simulink model "torqueBalancingJc_ikin_2012a"  (Simulink 8.0)
settings: Solver=FixedStepDiscrete  StartTime=0.0  StopTime=simulationTime  FixedStep=Ts  RelTol=1e-3
InitFcn:
  | initTorqueBalancingJc;
values from neighbouring files (symbols this model uses):
  LEFT_RIGHT_FOOT_IN_CONTACT = [1 1]    [initTorqueBalancingJc.m]
  localName = 'matlabTorqueBalancing'    [initTorqueBalancingJc.m]
  Ts = 0.01    [initTorqueBalancingJc.m]
undefined symbols (not defined in the file or in its folder): bVectorConstraints, ConstraintsMatrix, DiscIntNeverNeededParam, gain, reg, ROBOT_DOF, ROBOT_DOF_FOR_SIMULINK, sat
undefined symbols (not defined in the file): robotName
libraries: WBCLibrary x57, simulink x2
settings Model: Creator=daniele  LastModifiedBy=jorhabib
settings DebuggingCC: FcnCallInpInsideContextMsg=EnableAllAsWarning  FrameProcessingCompatibilityMsg=error
settings SFSimCC: SimParseCustomCode=off
settings CodeAppCC: CustomSymbolStrType=$N$R$M_T
settings GRTTargetCC: CodeReplacementLibrary=C89/C90 (ANSI)  CombineOutputUpdateFcns=off  GRTInterface=on

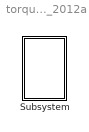
== system torqueBalancingJc_ikin_2012a ==
  Subsystem : Subsystem  mask{robotName=robotName, Ts=Ts, localName=localName}
      mask prompts: robotName "robot name"; localName "module name"

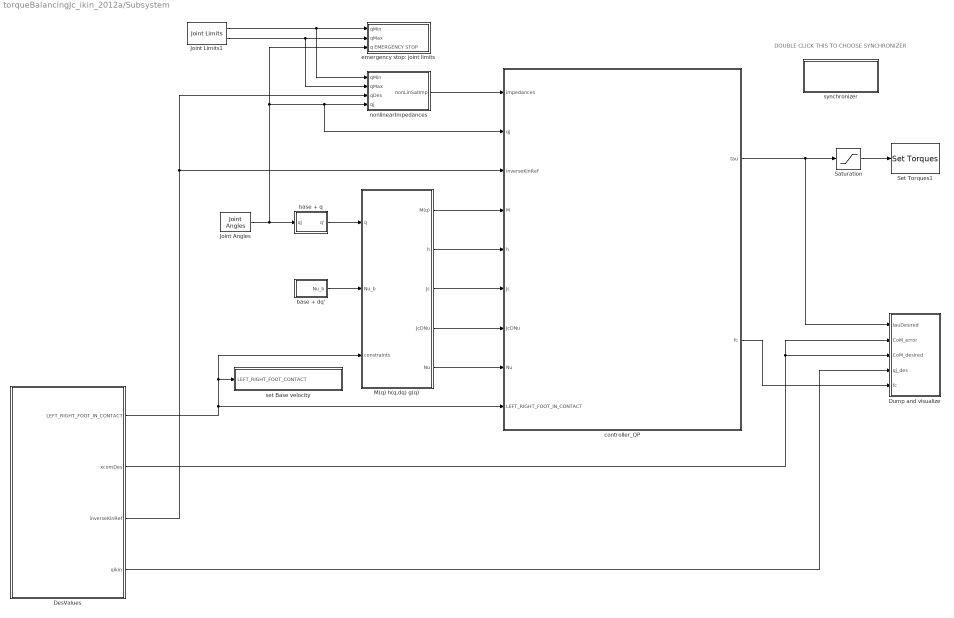
== system torqueBalancingJc_ikin_2012a/Subsystem ==
  note: DOUBLE CLICK THIS TO
      |  CHOOSE SYNCHRONIZER
  DesValues : Subsystem
  Dump and visualize : Subsystem
  Joint Angles : WBCLibrary/wholeBodyStates/Joint Angles  robotName=robotName  localName=localName
  Joint Limits1 : WBCLibrary/wholeBodyModel/Joint Limits  robotName=robotName  localName=localName
  M(q) h(q,dq) g(q) : Subsystem
  Saturation : Saturate  UpperLimit=sat.torque  LowerLimit=-sat.torque
  Set Torques1 : WBCLibrary/wholeBodyActuators/Set Torques  val=6  robotName=robotName  localName=localName
  base + dq' : Subsystem
  base + q : Subsystem
  controller_QP : Subsystem
  emergency stop: joint limits : Subsystem
  nonlinearImpedances : Subsystem
  set Base velocity : Subsystem  Description=Set base velocity
  synchronizer : Subsystem
  wires:
  base + q/1(q') -> M(q) h(q,dq) g(q)/1(q)
  M(q) h(q,dq) g(q)/1(M(q)) -> controller_QP/4(M)
  Joint Limits1/1 -> emergency stop: joint limits/1(qMin), nonlinearImpedances/1(qMin)
  Joint Limits1/2 -> emergency stop: joint limits/2(qMax), nonlinearImpedances/2(qMax)
  Joint Angles/1 -> emergency stop: joint limits/3(q EMERGENCY STOP), controller_QP/2(qj), nonlinearImpedances/4(qj), base + q/1(qj)
  M(q) h(q,dq) g(q)/2(h) -> controller_QP/5(h)
  controller_QP/1("tau ") -> Dump and visualize/1(tauDesired), Saturation/1
  Saturation/1 -> Set Torques1/1
  DesValues/1(LEFT_RIGHT_FOOT_IN_CONTACT) -> M(q) h(q,dq) g(q)/3(constraints), set Base velocity/1(LEFT_RIGHT_FOOT_CONTACT), controller_QP/9(LEFT_RIGHT_FOOT_IN_CONTACT)
  nonlinearImpedances/1(nonLinSatImp) -> controller_QP/1(impedances)
  M(q) h(q,dq) g(q)/5(Nu) -> controller_QP/8(Nu)
  M(q) h(q,dq) g(q)/3(Jc) -> controller_QP/6(Jc)
  M(q) h(q,dq) g(q)/4(JcDNu) -> controller_QP/7(JcDNu)
  DesValues/3(inverseKinRef) -> controller_QP/3(inverseKinRef), nonlinearImpedances/3(qDes)
  base + dq'/1(Nu_b) -> M(q) h(q,dq) g(q)/2(Nu_b)
  DesValues/4(qikin) -> Dump and visualize/4(qj_des)
  DesValues/2(xcomDes) -> Dump and visualize/2(CoM_error), Dump and visualize/3(CoM_desired)
  controller_QP/2(fc) -> Dump and visualize/5(fc)

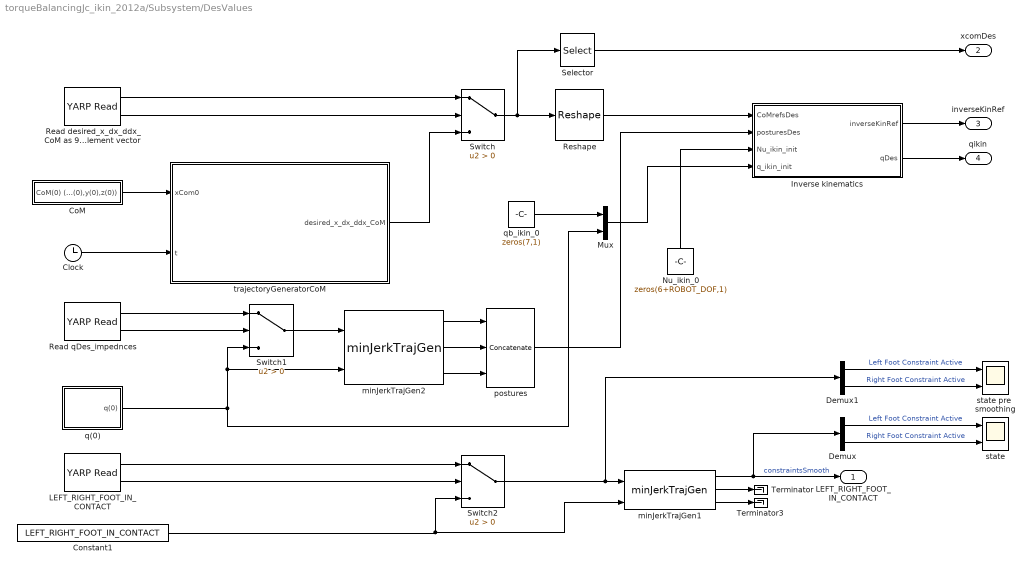
== system torqueBalancingJc_ikin_2012a/Subsystem/DesValues ==
  " LEFT_RIGHT_FOOT_IN_CONTACT" : WBCLibrary/Utilities/YARP Read  portName=['/' localName '/constraints:i']  signalSize=2  blocking=off  timestamp=off  autoconnect=off  errorOnConnection=on
  Clock : Clock
  "CoM " : Subsystem
  Constant1 : Constant  Value=LEFT_RIGHT_FOOT_IN_CONTACT
  Demux : Demux  Outputs=2
  Demux1 : Demux  Outputs=2
  Inverse kinematics : Subsystem
  Mux : Mux  Inputs=2
  Nu_ikin_0 : Constant  Value=zeros(6+ROBOT_DOF,1)
  "Read desired_x_dx_ddx_CoM as 9 element vector " : WBCLibrary/Utilities/YARP Read  portName=['/' localName '/comDes:i']  signalSize=9  blocking=off  timestamp=off  autoconnect=off  errorOnConnection=on
  Read qDes_impednces : WBCLibrary/Utilities/YARP Read  portName=['/' localName '/qDes:i']  signalSize=ROBOT_DOF  blocking=off  timestamp=off  autoconnect=off  errorOnConnection=on
  Reshape : Reshape  OutputDimensionality=Customize  OutputDimensions=[3,3]
  Selector : Selector  InputPortWidth=9  IndexOptions=Index vector (dialog)  Indices=[1:3]  OutputSizes=1
  Switch : Switch  Criteria=u2 > Threshold
  Switch1 : Switch  Criteria=u2 > Threshold
  Switch2 : Switch  Criteria=u2 > Threshold
  Terminator : Terminator
  Terminator3 : Terminator
  minJerkTrajGen1 : WBCLibrary/Utilities/minJerkTrajGen  dim=2  Ts=Ts  Tt=smoothingTimeJacobians
  minJerkTrajGen2 : WBCLibrary/Utilities/minJerkTrajGen  dim=ROBOT_DOF  Ts=Ts  Tt=smoothingTimePostures
  postures : Concatenate  NumInputs=3  Mode=Multidimensional array  ConcatenateDimension=2
  q(0) : Subsystem
  qb_ikin_0 : Constant  Value=zeros(7,1)
  state : Scope  NumInputPorts=2
      settings: ShowLegends=on  TimeRange=60  YMin=0~0  YMax=2~2
  state pre  smoothing : Scope  NumInputPorts=2
      settings: ShowLegends=on  TimeRange=60  YMin=0~0  YMax=2~2  SaveName=ScopeData7
  trajectoryGeneratorCoM : MATLAB Function  TreatAsAtomicUnit=on
  LEFT_RIGHT_FOOT_IN_CONTACT : Outport
  xcomDes : Outport  Port=2
  inverseKinRef : Outport  Port=3
  qikin : Outport  Port=4
  wires:
  Constant1/1 -> Switch2/3, minJerkTrajGen1/2
  minJerkTrajGen1/1 -> Demux/1, LEFT_RIGHT_FOOT_IN_CONTACT/1  "constraintsSmooth"
  minJerkTrajGen1/2 -> Terminator/1
  minJerkTrajGen1/3 -> Terminator3/1
  "Read desired_x_dx_ddx_CoM as 9 element vector "/2 -> Switch/2
  "Read desired_x_dx_ddx_CoM as 9 element vector "/1 -> Switch/1
  Reshape/1 -> Inverse kinematics/1(CoMrefsDes)
  Switch/1 -> Selector/1, Reshape/1
  Read qDes_impednces/2 -> Switch1/2
  Read qDes_impednces/1 -> Switch1/1
  Selector/1 -> xcomDes/1
  " LEFT_RIGHT_FOOT_IN_CONTACT"/2 -> Switch2/2
  " LEFT_RIGHT_FOOT_IN_CONTACT"/1 -> Switch2/1
  Switch2/1 -> Demux1/1, minJerkTrajGen1/1
  Demux/1 -> state/1  "Left Foot Constraint Active"
  Demux/2 -> state/2  "Right Foot Constraint Active"
  Demux1/1 -> state pre  smoothing/1  "Left Foot Constraint Active"
  Demux1/2 -> state pre  smoothing/2  "Right Foot Constraint Active"
  "CoM "/1(CoM(0) (x(0),y(0),z(0))) -> trajectoryGeneratorCoM/1(xCom0)
  Clock/1 -> trajectoryGeneratorCoM/2(t)
  trajectoryGeneratorCoM/1(desired_x_dx_ddx_CoM) -> Switch/3
  Switch1/1 -> minJerkTrajGen2/1
  minJerkTrajGen2/1 -> postures/1
  minJerkTrajGen2/2 -> postures/2
  minJerkTrajGen2/3 -> postures/3
  Nu_ikin_0/1 -> Inverse kinematics/3(Nu_ikin_init)
  qb_ikin_0/1 -> Mux/1
  Mux/1 -> Inverse kinematics/4(q_ikin_init)
  q(0)/1(q(0)) -> Mux/2, Switch1/3, minJerkTrajGen2/2
  Inverse kinematics/1(inverseKinRef) -> inverseKinRef/1
  postures/1 -> Inverse kinematics/2(posturesDes)
  Inverse kinematics/2(qDes) -> qikin/1

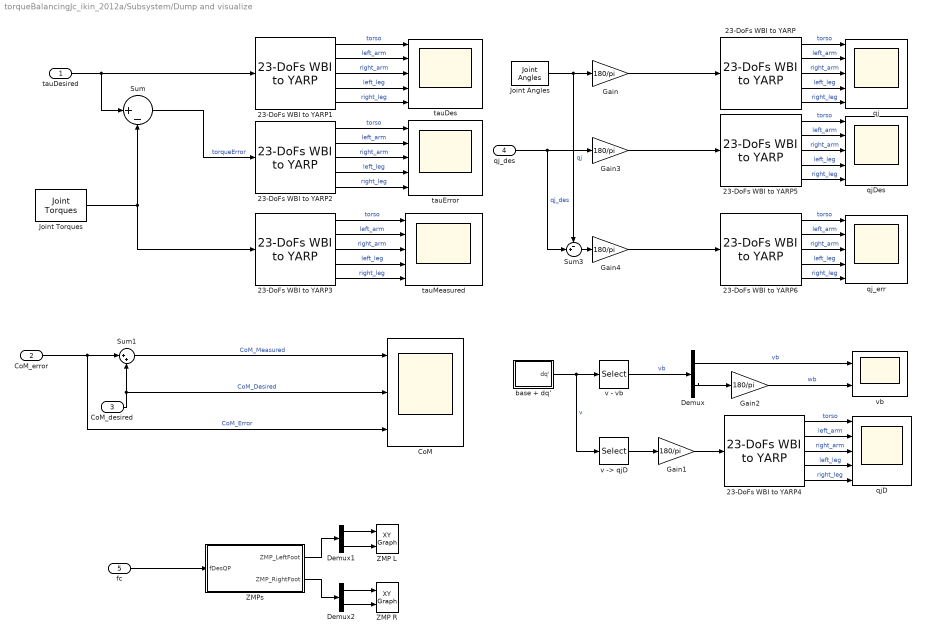
== system torqueBalancingJc_ikin_2012a/Subsystem/Dump and visualize ==
  tauDesired : Inport
  CoM_error : Inport  Port=2
  CoM_desired : Inport  Port=3
  qj_des : Inport  Port=4
  fc : Inport  Port=5
  23-DoFs WBI to YARP{,1..6} (7 alike) : WBCLibrary/Utilities/23-DoFs WBI to YARP
  CoM : Scope  NumInputPorts=3
      settings: ShowLegends=on  TimeRange=400  YMin=-0.2~-0.2~-0.006  YMax=0.5~0.5~0.004  SaveName=CoM_data
  Demux : Demux  Outputs=2
  Demux1 : Demux  Outputs=2
  Demux2 : Demux  Outputs=2
  Gain{,1..4} (5 alike) : Gain  Gain=180/pi
  Joint Angles : WBCLibrary/wholeBodyStates/Joint Angles  robotName=robotName  localName=localName
  Joint Torques : WBCLibrary/wholeBodyStates/Joint Torques  robotName=robotName  localName=localName
  Sum : Sum  Inputs=|+-
  Sum1 : Sum  Inputs=|++
  Sum3 : Sum  Inputs=-+|
  ZMP L : simulink/Sinks/XY Graph  xmin=gain.footSize(1,1)  xmax=gain.footSize(1,2)  ymin=gain.footSize(2,1)  ymax=gain.footSize(2,2)  st=-1
  ZMP R : simulink/Sinks/XY Graph  xmin=gain.footSize(1,1)  xmax=gain.footSize(1,2)  ymin=gain.footSize(2,1)  ymax=gain.footSize(2,2)  st=-1
  ZMPs : Subsystem
  base + dq' : Subsystem
  qj : Scope  NumInputPorts=5
      settings: ShowLegends=on  TimeRange=40  YMin=-6~-40~-40~-15~-10  YMax=2~60~60~15~12.5  SaveName=qj_and_v
  qjD : Scope  NumInputPorts=5
      settings: ShowLegends=on  TimeRange=40  YMin=-15~-10~-20~-20~-20  YMax=20~10~30~20~20  SaveName=qj_and_v1
  qjDes : Scope  NumInputPorts=5
      settings: ShowLegends=on  TimeRange=40  YMin=-6~-40~-40~-15~-10  YMax=2~60~60~15~12.5  SaveName=qj_and_v3
  qj_err : Scope  NumInputPorts=5
      settings: ShowLegends=on  TimeRange=40  YMin=-0.05~-0.01~-0.015~-0.25~-0.5  YMax=0.125~0.02~0.02~1.25~2.5  SaveName=qj_and_v4
  tauDes : Scope  NumInputPorts=5
      settings: ShowLegends=on  TimeRange=14  YMin=-5~-2.5~-2.5~-4~-3.5  YMax=1~1.5~1.5~3~2  SaveName=tauDes
  tauError : Scope  NumInputPorts=5
      settings: ShowLegends=on  TimeRange=90  YMin=-3.94704~-2.86095~-2.77437~-5.99629~-4.78678  YMax=3.1474~3.19748~2.86308~6.73695~4.3906  SaveName=tauError
  tauMeasured : Scope  NumInputPorts=5
      settings: ShowLegends=on  TimeRange=14  YMin=-800000~-300000~-300000~-500000~-1e+06  YMax=100000~200000~200000~600000~1e+06  SaveName=tauMeasured
  v - vb : Selector  InputPortWidth=ROBOT_DOF+6  IndexOptions=Index vector (dialog)  Indices=[1:6]  OutputSizes=1
  "v -> qjD" : Selector  InputPortWidth=ROBOT_DOF+6  IndexOptions=Index vector (dialog)  Indices=[7:ROBOT_DOF+6]  OutputSizes=1
  vb : Scope  NumInputPorts=2
      settings: ShowLegends=on  TimeRange=40  YMin=-0.08~-10  YMax=0.08~10  SaveName=qj_and_v2
  wires:
  CoM_error/1 -> CoM/3, Sum1/1  "CoM_Error"
  CoM_desired/1 -> Sum1/2, CoM/2  "CoM_Desired"
  Sum1/1 -> CoM/1  "CoM_Measured"
  base + dq'/1(dq') -> "v -> qjD"/1, v - vb/1  "v"
  Joint Angles/1 -> Sum3/1, Gain/1  "qj"
  Gain/1 -> 23-DoFs WBI to YARP/1
  23-DoFs WBI to YARP/5 -> qj/5  "right_leg"
  23-DoFs WBI to YARP/1 -> qj/1  "torso"
  23-DoFs WBI to YARP/2 -> qj/2  "left_arm"
  23-DoFs WBI to YARP/4 -> qj/4  "left_leg"
  23-DoFs WBI to YARP/3 -> qj/3  "right_arm"
  23-DoFs WBI to YARP4/5 -> qjD/5  "right_leg"
  23-DoFs WBI to YARP4/1 -> qjD/1  "torso"
  23-DoFs WBI to YARP4/2 -> qjD/2  "left_arm"
  23-DoFs WBI to YARP4/4 -> qjD/4  "left_leg"
  23-DoFs WBI to YARP4/3 -> qjD/3  "right_arm"
  "v -> qjD"/1 -> Gain1/1
  v - vb/1 -> Demux/1  "vb"
  Demux/1 -> vb/1  "vb"
  Demux/2 -> Gain2/1
  Gain1/1 -> 23-DoFs WBI to YARP4/1
  Gain2/1 -> vb/2  "wb"
  fc/1 -> ZMPs/1(fDesQP)
  ZMPs/1(ZMP_LeftFoot) -> Demux1/1
  ZMPs/2(ZMP_RightFoot) -> Demux2/1
  Demux1/1 -> ZMP L/1
  Demux1/2 -> ZMP L/2
  Demux2/1 -> ZMP R/1
  Demux2/2 -> ZMP R/2
  tauDesired/1 -> Sum/1, 23-DoFs WBI to YARP1/1
  Joint Torques/1 -> 23-DoFs WBI to YARP3/1, Sum/2
  23-DoFs WBI to YARP1/5 -> tauDes/5  "right_leg"
  23-DoFs WBI to YARP1/1 -> tauDes/1  "torso"
  23-DoFs WBI to YARP1/2 -> tauDes/2  "left_arm"
  23-DoFs WBI to YARP1/4 -> tauDes/4  "left_leg"
  23-DoFs WBI to YARP1/3 -> tauDes/3  "right_arm"
  23-DoFs WBI to YARP2/5 -> tauError/5  "right_leg"
  23-DoFs WBI to YARP2/1 -> tauError/1  "torso"
  23-DoFs WBI to YARP2/2 -> tauError/2  "left_arm"
  23-DoFs WBI to YARP2/4 -> tauError/4  "left_leg"
  23-DoFs WBI to YARP2/3 -> tauError/3  "right_arm"
  Sum/1 -> 23-DoFs WBI to YARP2/1  "torqueError"
  23-DoFs WBI to YARP3/5 -> tauMeasured/5  "right_leg"
  23-DoFs WBI to YARP3/1 -> tauMeasured/1  "torso"
  23-DoFs WBI to YARP3/2 -> tauMeasured/2  "left_arm"
  23-DoFs WBI to YARP3/4 -> tauMeasured/4  "left_leg"
  23-DoFs WBI to YARP3/3 -> tauMeasured/3  "right_arm"
  Gain3/1 -> 23-DoFs WBI to YARP5/1
  23-DoFs WBI to YARP5/5 -> qjDes/5  "right_leg"
  23-DoFs WBI to YARP5/1 -> qjDes/1  "torso"
  23-DoFs WBI to YARP5/2 -> qjDes/2  "left_arm"
  23-DoFs WBI to YARP5/4 -> qjDes/4  "left_leg"
  23-DoFs WBI to YARP5/3 -> qjDes/3  "right_arm"
  Gain4/1 -> 23-DoFs WBI to YARP6/1
  23-DoFs WBI to YARP6/5 -> qj_err/5  "right_leg"
  23-DoFs WBI to YARP6/1 -> qj_err/1  "torso"
  23-DoFs WBI to YARP6/2 -> qj_err/2  "left_arm"
  23-DoFs WBI to YARP6/4 -> qj_err/4  "left_leg"
  23-DoFs WBI to YARP6/3 -> qj_err/3  "right_arm"
  Sum3/1 -> Gain4/1
  qj_des/1 -> Gain3/1, Sum3/2  "qj_des"

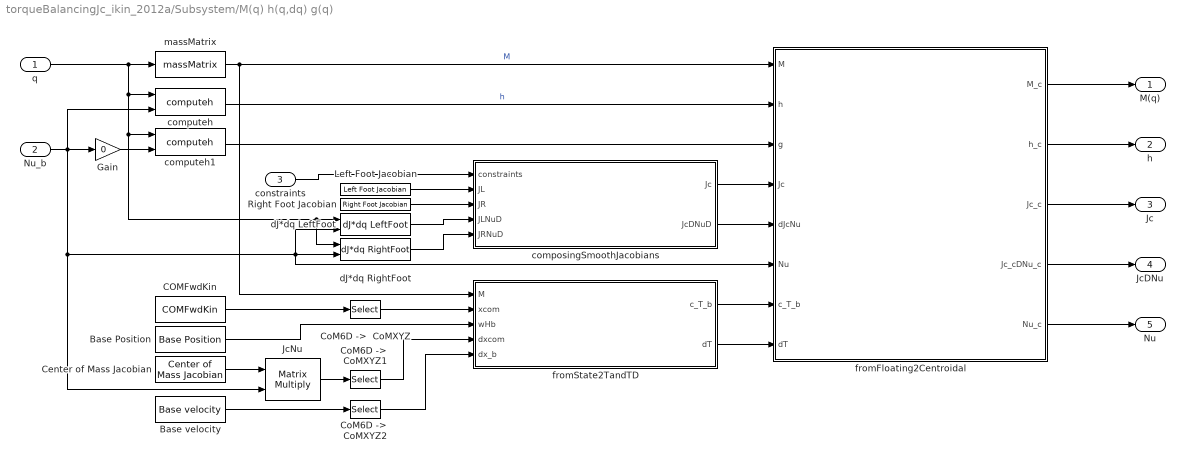
== system torqueBalancingJc_ikin_2012a/Subsystem/M(q) h(q,dq) g(q) ==
  q : Inport
  Nu_b : Inport  Port=2
  constraints : Inport  Port=3
  Base Position : WBCLibrary/wholeBodyStates/Base Position  robotName=robotName  localName=localName
  Base velocity : WBCLibrary/wholeBodyStates/Base velocity  robotName=robotName  localName=localName
  "COMFwdKin " : WBCLibrary/wholeBodyModel/Forward Kinematics/COMFwdKin   robotName=robotName  localName=localName
  Center of Mass Jacobian : WBCLibrary/wholeBodyModel/Jacobians/Center of Mass Jacobian  robotName=robotName  localName=localName
  "CoM6D ->  CoMXYZ" : Selector  InputPortWidth=7  IndexOptions=Index vector (dialog)  Indices=[1 2 3]  OutputSizes=1
  "CoM6D ->  CoMXYZ1" : Selector  InputPortWidth=6  IndexOptions=Index vector (dialog)  Indices=[1 2 3]  OutputSizes=1
  "CoM6D ->  CoMXYZ2" : Selector  InputPortWidth=6  IndexOptions=Index vector (dialog)  Indices=[1 2 3]  OutputSizes=1
  Gain : Gain  Gain=0
  JcNu : Product  Multiplication=Matrix(*)
  Left Foot Jacobian : WBCLibrary/wholeBodyModel/Jacobians/Left Foot Jacobian  robotName=robotName  localName=localName
  Right Foot Jacobian : WBCLibrary/wholeBodyModel/Jacobians/Right Foot Jacobian  robotName=robotName  localName=localName
  composingSmoothJacobians : MATLAB Function  TreatAsAtomicUnit=on
  computeh : WBCLibrary/wholeBodyModel/Dynamics/computeh  val=7  robotname=robotName  localname=localName
  computeh1 : WBCLibrary/wholeBodyModel/Dynamics/computeh  val=7  robotname=robotName  localname=localName
  dJ*dq LeftFoot : WBCLibrary/wholeBodyModel/Dynamics/dJ*dq LeftFoot  val=9  robotName=robotName  localName=localName
  dJ*dq RightFoot : WBCLibrary/wholeBodyModel/Dynamics/dJ*dq RightFoot  val=9  robotName=robotName  localName=localName
  fromFloating2Centroidal : MATLAB Function  TreatAsAtomicUnit=on
  fromState2TandTD : MATLAB Function  TreatAsAtomicUnit=on
  massMatrix : WBCLibrary/wholeBodyModel/Dynamics/massMatrix  val=8  robotname=robotName  localname=localName
  M(q) : Outport
  h : Outport  Port=2
  Jc : Outport  Port=3
  JcDNu : Outport  Port=4
  Nu : Outport  Port=5
  wires:
  q/1 -> computeh1/1, dJ*dq RightFoot/1, dJ*dq LeftFoot/1, computeh/1, massMatrix/1
  Nu_b/1 -> Gain/1, computeh/2, fromFloating2Centroidal/6(Nu), dJ*dq LeftFoot/2, dJ*dq RightFoot/2, JcNu/2
  Gain/1 -> computeh1/2
  massMatrix/1 -> fromFloating2Centroidal/1(M), fromState2TandTD/1(M)  "M"
  fromState2TandTD/1(c_T_b) -> fromFloating2Centroidal/7(c_T_b)
  fromState2TandTD/2(dT) -> fromFloating2Centroidal/8(dT)
  computeh/1 -> fromFloating2Centroidal/2(h)  "h"
  computeh1/1 -> fromFloating2Centroidal/3(g)
  "COMFwdKin "/1 -> "CoM6D ->  CoMXYZ"/1
  "CoM6D ->  CoMXYZ"/1 -> fromState2TandTD/2(xcom)
  Base velocity/1 -> "CoM6D ->  CoMXYZ2"/1
  "CoM6D ->  CoMXYZ2"/1 -> fromState2TandTD/5(dx_b)
  Base Position/1 -> fromState2TandTD/3(wHb)
  Center of Mass Jacobian/1 -> JcNu/1
  JcNu/1 -> "CoM6D ->  CoMXYZ1"/1
  "CoM6D ->  CoMXYZ1"/1 -> fromState2TandTD/4(dxcom)
  composingSmoothJacobians/1(Jc) -> fromFloating2Centroidal/4(Jc)
  composingSmoothJacobians/2(JcDNuD) -> fromFloating2Centroidal/5(dJcNu)
  constraints/1 -> composingSmoothJacobians/1(constraints)
  Left Foot Jacobian/1 -> composingSmoothJacobians/2(JL)
  Right Foot Jacobian/1 -> composingSmoothJacobians/3(JR)
  dJ*dq LeftFoot/1 -> composingSmoothJacobians/4(JLNuD)
  dJ*dq RightFoot/1 -> composingSmoothJacobians/5(JRNuD)
  fromFloating2Centroidal/1(M_c) -> M(q)/1
  fromFloating2Centroidal/2(h_c) -> h/1
  fromFloating2Centroidal/3(Jc_c) -> Jc/1
  fromFloating2Centroidal/4(Jc_cDNu_c) -> JcDNu/1
  fromFloating2Centroidal/5(Nu_c) -> Nu/1

== system torqueBalancingJc_ikin_2012a/Subsystem/base + dq' ==
  Base velocity : WBCLibrary/wholeBodyStates/Base velocity  robotName=robotName  localName=localName
  Joint Velocities : WBCLibrary/wholeBodyStates/Joint Velocities  robotName=robotName  localName=localName
  Mux : Mux  Inputs=2
  Nu_b : Outport
  wires:
  Base velocity/1 -> Mux/1
  Joint Velocities/1 -> Mux/2
  Mux/1 -> Nu_b/1

== system torqueBalancingJc_ikin_2012a/Subsystem/base + q ==
  qj : Inport
  Constant1 : Constant  Value=zeros(16,1)
  Mux : Mux  Inputs=2
  q' : Outport
  wires:
  Mux/1 -> q'/1
  qj/1 -> Mux/2
  Constant1/1 -> Mux/1

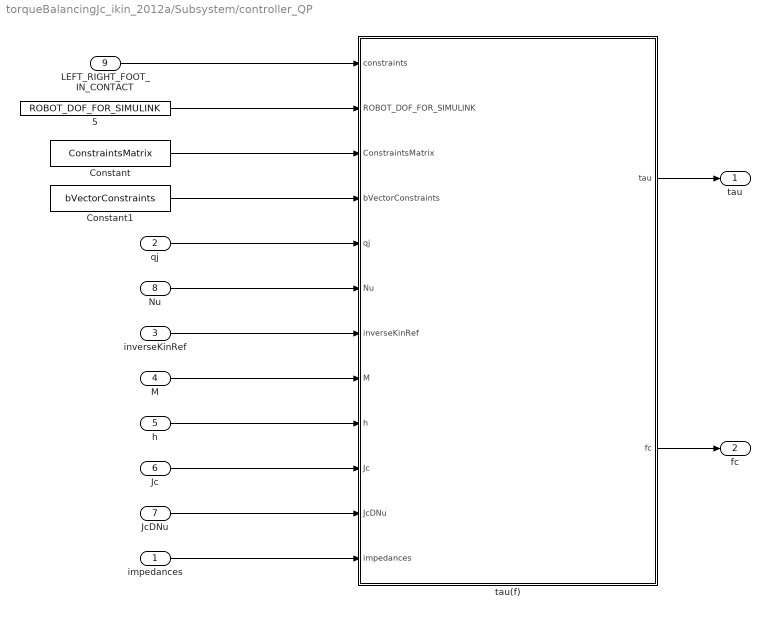
== system torqueBalancingJc_ikin_2012a/Subsystem/controller_QP ==
  impedances : Inport
  qj : Inport  Port=2
  inverseKinRef : Inport  Port=3
  M : Inport  Port=4
  h : Inport  Port=5
  Jc : Inport  Port=6
  JcDNu : Inport  Port=7
  Nu : Inport  Port=8
  LEFT_RIGHT_FOOT_IN_CONTACT : Inport  Port=9
  "    5" : Constant  Value=ROBOT_DOF_FOR_SIMULINK
  Constant : Constant  Value=ConstraintsMatrix
  Constant1 : Constant  Value=bVectorConstraints
  "tau(f) " : MATLAB Function  TreatAsAtomicUnit=on
  "tau " : Outport
  fc : Outport  Port=2
  wires:
  LEFT_RIGHT_FOOT_IN_CONTACT/1 -> "tau(f) "/1(constraints)
  M/1 -> "tau(f) "/8(M)
  h/1 -> "tau(f) "/9(h)
  "    5"/1 -> "tau(f) "/2(ROBOT_DOF_FOR_SIMULINK)
  Constant/1 -> "tau(f) "/3(ConstraintsMatrix)
  Constant1/1 -> "tau(f) "/4(bVectorConstraints)
  Jc/1 -> "tau(f) "/10(Jc)
  JcDNu/1 -> "tau(f) "/11(JcDNu)
  Nu/1 -> "tau(f) "/6(Nu)
  impedances/1 -> "tau(f) "/12(impedances)
  "tau(f) "/1(tau) -> "tau "/1
  qj/1 -> "tau(f) "/5(qj)
  inverseKinRef/1 -> "tau(f) "/7(inverseKinRef)
  "tau(f) "/2(fc) -> fc/1

== system torqueBalancingJc_ikin_2012a/Subsystem/emergency stop: joint limits ==
  qMin : Inport
  qMax : Inport  Port=2
  q EMERGENCY STOP : Inport  Port=3
  Assertion : Assertion  Enabled=on
  MATLAB Function : MATLAB Function  TreatAsAtomicUnit=on
  index1 : Constant  Value=0.01  VectorParams1D=off
  wires:
  qMin/1 -> MATLAB Function/1(umin)
  qMax/1 -> MATLAB Function/2(umax)
  index1/1 -> MATLAB Function/4(tol)
  q EMERGENCY STOP/1 -> MATLAB Function/3(u)
  MATLAB Function/1(inRange) -> Assertion/1

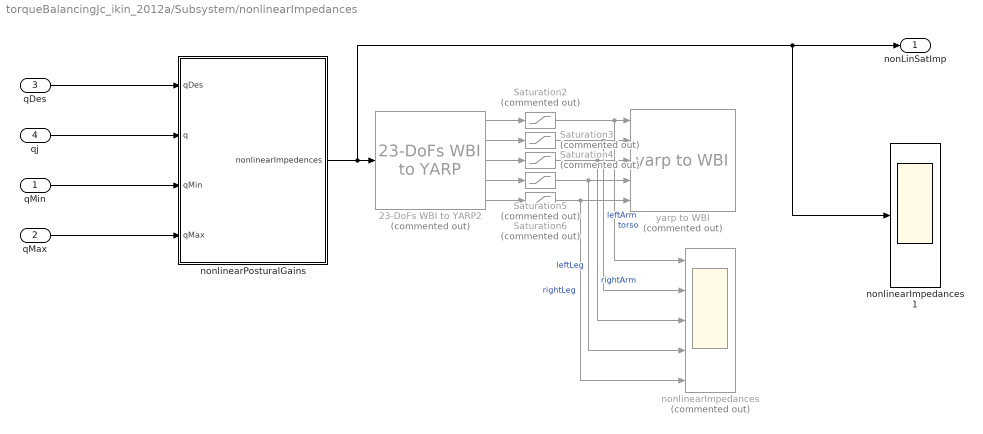
== system torqueBalancingJc_ikin_2012a/Subsystem/nonlinearImpedances ==
  qMin : Inport
  qMax : Inport  Port=2
  qDes : Inport  Port=3
  qj : Inport  Port=4
  23-DoFs WBI to YARP2 : WBCLibrary/Utilities/23-DoFs WBI to YARP  Commented=on
  Saturation2 : Saturate  Commented=on  UpperLimit=sat.impedences(1)  LowerLimit=0  SampleTime=Ts
  Saturation3 : Saturate  Commented=on  UpperLimit=sat.impedences(2)  LowerLimit=0  SampleTime=Ts
  Saturation4 : Saturate  Commented=on  UpperLimit=sat.impedences(2)  LowerLimit=0  SampleTime=Ts
  Saturation5 : Saturate  Commented=on  UpperLimit=sat.impedences(3)  LowerLimit=0  SampleTime=Ts
  Saturation6 : Saturate  Commented=on  UpperLimit=sat.impedences(3)  LowerLimit=0  SampleTime=Ts
  nonlinearImpedances : Scope  Commented=on  NumInputPorts=5
      settings: ShowLegends=on  TimeRange=25  YMin=-50~-50~-50~0~0  YMax=50~50~50~1000~1000
  nonlinearImpedances1 : Scope
      settings: ShowLegends=on  TimeRange=25  YMin=-50  YMax=50
  "nonlinearPosturalGains " : MATLAB Function  TreatAsAtomicUnit=on
  yarp to WBI : WBCLibrary/Utilities/yarp to WBI  Commented=on
  nonLinSatImp : Outport
  wires:
  23-DoFs WBI to YARP2/1 -> Saturation2/1
  23-DoFs WBI to YARP2/2 -> Saturation3/1
  23-DoFs WBI to YARP2/3 -> Saturation4/1
  23-DoFs WBI to YARP2/5 -> Saturation6/1
  "nonlinearPosturalGains "/1(nonlinearImpedences) -> nonlinearImpedances1/1, nonLinSatImp/1, 23-DoFs WBI to YARP2/1
  qMin/1 -> "nonlinearPosturalGains "/3(qMin)
  qMax/1 -> "nonlinearPosturalGains "/4(qMax)
  qj/1 -> "nonlinearPosturalGains "/2(q)
  Saturation6/1 -> nonlinearImpedances/5, yarp to WBI/5  "rightLeg"
  Saturation4/1 -> nonlinearImpedances/3, yarp to WBI/3  "rightArm"
  Saturation5/1 -> nonlinearImpedances/4, yarp to WBI/4  "leftLeg"
  Saturation3/1 -> nonlinearImpedances/2, yarp to WBI/2  "leftArm"
  Saturation2/1 -> nonlinearImpedances/1, yarp to WBI/1  "torso"
  23-DoFs WBI to YARP2/4 -> Saturation5/1
  qDes/1 -> "nonlinearPosturalGains "/1(qDes)

== system torqueBalancingJc_ikin_2012a/Subsystem/set Base velocity ==
  LEFT_RIGHT_FOOT_CONTACT : Inport
  Joint Velocities : WBCLibrary/wholeBodyStates/Joint Velocities  robotName=robotName  localName=localName
  Left Foot Jacobian : WBCLibrary/wholeBodyModel/Jacobians/Left Foot Jacobian  robotName=robotName  localName=localName
  Right Foot Jacobian : WBCLibrary/wholeBodyModel/Jacobians/Right Foot Jacobian  robotName=robotName  localName=localName
  Set base velocity (w.r.t. world) : WBCLibrary/wholeBodyStates/Set base velocity (w.r.t. world)  Priority=-1  robotName=robotName  localName=localName
  baseVelocity : Subsystem  AncestorBlock=WBCLibrary/Utilities/baseVelocity  mask(baseVelocity){}
      mask help: This block computes the velocity of the floating base of a bipedal robot
  wires:
  Left Foot Jacobian/1 -> baseVelocity/2(JacobLF)
  Right Foot Jacobian/1 -> baseVelocity/1(JacobRF)
  baseVelocity/1(baseVel) -> Set base velocity (w.r.t. world)/1
  Joint Velocities/1 -> baseVelocity/3(dq)
  LEFT_RIGHT_FOOT_CONTACT/1 -> baseVelocity/4(LEFT_RIGHT_FOOT_CONTACT)

== system torqueBalancingJc_ikin_2012a/Subsystem/synchronizer ==
  Real Time Synchronizer : WBCLibrary/Utilities/Real Time Synchronizer  Commented=on  threadPeriod=Ts
  synchronize : WBCLibrary/Utilities/synchronize  rate=0.010  scaleFactor=1

== system torqueBalancingJc_ikin_2012a/Subsystem/DesValues/CoM  ==
  "COMFwdKin " : WBCLibrary/wholeBodyModel/Forward Kinematics/COMFwdKin   robotName=robotName  localName=localName
  "CoM6D ->  CoMXYZ" : Selector  InputPortWidth=7  IndexOptions=Index vector (dialog)  Indices=[1 2 3]  OutputSizes=1
  "holder " : WBCLibrary/Utilities/holder 
  CoM(0) (x(0),y(0),z(0)) : Outport
  wires:
  "COMFwdKin "/1 -> "CoM6D ->  CoMXYZ"/1
  "CoM6D ->  CoMXYZ"/1 -> "holder "/1
  "holder "/1 -> CoM(0) (x(0),y(0),z(0))/1

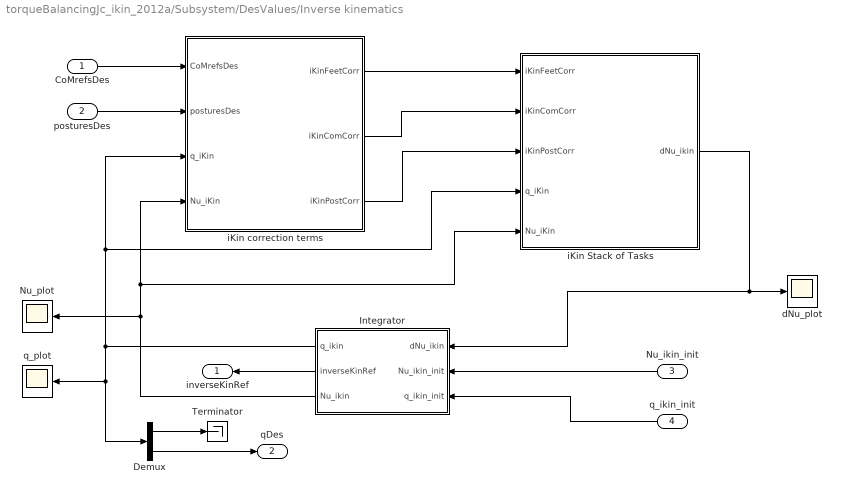
== system torqueBalancingJc_ikin_2012a/Subsystem/DesValues/Inverse kinematics ==
  CoMrefsDes : Inport
  posturesDes : Inport  Port=2
  Nu_ikin_init : Inport  Port=3
  q_ikin_init : Inport  Port=4
  Demux : Demux  Outputs=[16;ROBOT_DOF]
  Integrator : Subsystem
  Nu_plot : Scope
      settings: TimeRange=10  YMin=-0.00125  YMax=0.002  SaveName=ScopeData3
  Terminator : Terminator
  dNu_plot : Scope
      settings: YMin=-0.007  YMax=0.007  SaveName=ScopeData2
  iKin Stack of Tasks : Subsystem
  iKin correction terms : Subsystem
  q_plot : Scope
      settings: YMin=-0.75  YMax=1  SaveName=ScopeData4
  inverseKinRef : Outport
  qDes : Outport  Port=2
  wires:
  CoMrefsDes/1 -> iKin correction terms/1(CoMrefsDes)
  posturesDes/1 -> iKin correction terms/2(posturesDes)
  iKin correction terms/1(iKinFeetCorr) -> iKin Stack of Tasks/1(iKinFeetCorr)
  iKin correction terms/2(iKinComCorr) -> iKin Stack of Tasks/2(iKinComCorr)
  iKin correction terms/3(iKinPostCorr) -> iKin Stack of Tasks/3(iKinPostCorr)
  Integrator/1(q_ikin) -> iKin correction terms/3(q_iKin), iKin Stack of Tasks/4(q_iKin), q_plot/1, Demux/1
  Nu_ikin_init/1 -> Integrator/2(Nu_ikin_init)
  q_ikin_init/1 -> Integrator/3(q_ikin_init)
  Integrator/2(inverseKinRef) -> inverseKinRef/1
  Integrator/3(Nu_ikin) -> Nu_plot/1, iKin correction terms/4(Nu_iKin), iKin Stack of Tasks/5(Nu_iKin)
  iKin Stack of Tasks/1(dNu_ikin) -> Integrator/1(dNu_ikin), dNu_plot/1
  Demux/2 -> qDes/1
  Demux/1 -> Terminator/1

== system torqueBalancingJc_ikin_2012a/Subsystem/DesValues/q(0) ==
  Joint Angles : WBCLibrary/wholeBodyStates/Joint Angles  robotName=robotName  localName=localName
  holder 1 : WBCLibrary/Utilities/holder 
  q(0) : Outport
  wires:
  Joint Angles/1 -> holder 1/1
  holder 1/1 -> q(0)/1

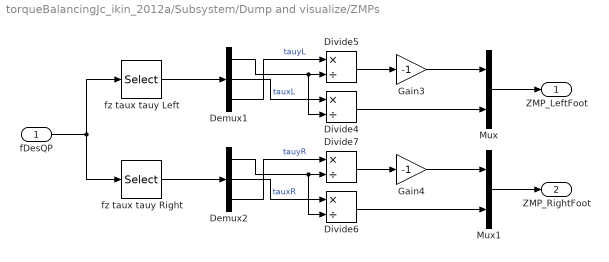
== system torqueBalancingJc_ikin_2012a/Subsystem/Dump and visualize/ZMPs ==
  fDesQP : Inport
  Demux1 : Demux  Outputs=3
  Demux2 : Demux  Outputs=3
  Divide{4..7} (4 alike) : Product  Inputs=*/
  Gain3 : Gain  Gain=-1
  Gain4 : Gain  Gain=-1
  Mux : Mux  Inputs=2
  Mux1 : Mux  Inputs=2
  fz taux tauy Left : Selector  InputPortWidth=12  IndexOptions=Index vector (dialog)  Indices=[3 4 5]  OutputSizes=1
  fz taux tauy Right : Selector  InputPortWidth=12  IndexOptions=Index vector (dialog)  Indices=[9 10 11]  OutputSizes=1
  ZMP_LeftFoot : Outport
  ZMP_RightFoot : Outport  Port=2
  wires:
  fz taux tauy Left/1 -> Demux1/1
  Demux1/1 -> Divide4/2, Divide5/2
  Divide7/1 -> Gain4/1
  Divide4/1 -> Mux/2
  Divide5/1 -> Gain3/1
  fz taux tauy Right/1 -> Demux2/1
  Demux2/1 -> Divide6/2, Divide7/2
  fDesQP/1 -> fz taux tauy Left/1, fz taux tauy Right/1
  Gain3/1 -> Mux/1
  Mux/1 -> ZMP_LeftFoot/1
  Divide6/1 -> Mux1/2
  Gain4/1 -> Mux1/1
  Mux1/1 -> ZMP_RightFoot/1
  Demux1/2 -> Divide4/1  "tauxL"
  Demux1/3 -> Divide5/1  "tauyL"
  Demux2/2 -> Divide6/1  "tauxR"
  Demux2/3 -> Divide7/1  "tauyR"

== system torqueBalancingJc_ikin_2012a/Subsystem/Dump and visualize/base + dq' ==
  Joint Velocities : WBCLibrary/wholeBodyStates/Joint Velocities  robotName=robotName  localName=localName
  Left Foot Jacobian : WBCLibrary/wholeBodyModel/Jacobians/Left Foot Jacobian  robotName=robotName  localName=localName
  Mux : Mux  Inputs=2
  Right Foot Jacobian : WBCLibrary/wholeBodyModel/Jacobians/Right Foot Jacobian  robotName=robotName  localName=localName
  baseVelocity : Subsystem  AncestorBlock=WBCLibrary/Utilities/baseVelocity  mask(baseVelocity){}
      mask help: This block computes the velocity of the floating base of a bipedal robot
  dq' : Outport
  wires:
  Left Foot Jacobian/1 -> baseVelocity/2(JacobLF)
  Right Foot Jacobian/1 -> baseVelocity/1(JacobRF)
  baseVelocity/1(baseVel) -> Mux/1
  Joint Velocities/1 -> baseVelocity/3(dq), Mux/2
  Mux/1 -> dq'/1

== system torqueBalancingJc_ikin_2012a/Subsystem/set Base velocity/baseVelocity ==
  JacobRF : Inport
  JacobLF : Inport  Port=2
  dq : Inport  Port=3
  LEFT_RIGHT_FOOT_CONTACT : Inport  Port=4
  MATLAB Function : MATLAB Function  TreatAsAtomicUnit=on
  baseVel : Outport
  wires:
  JacobLF/1 -> MATLAB Function/1(JcLeftFoot)
  JacobRF/1 -> MATLAB Function/2(JcRightFoot)
  MATLAB Function/1(y) -> baseVel/1
  dq/1 -> MATLAB Function/4(qD)
  LEFT_RIGHT_FOOT_CONTACT/1 -> MATLAB Function/3(activeFeetConstraints)

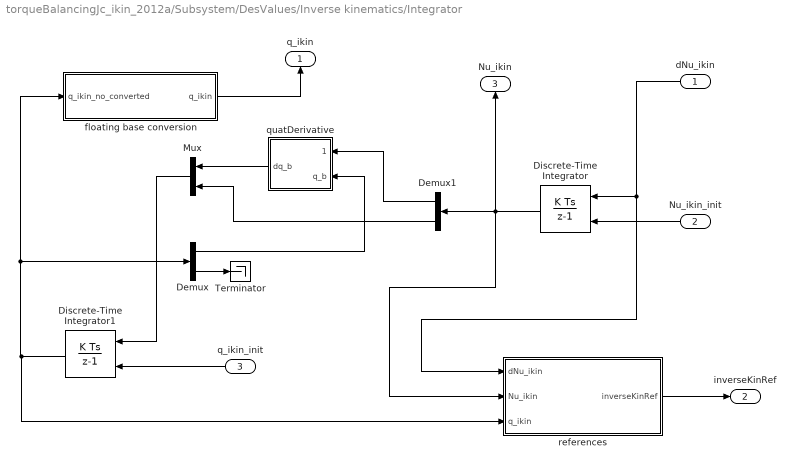
== system torqueBalancingJc_ikin_2012a/Subsystem/DesValues/Inverse kinematics/Integrator ==
  dNu_ikin : Inport
  Nu_ikin_init : Inport  Port=2
  q_ikin_init : Inport  Port=3
  Demux : Demux  Outputs=[7;ROBOT_DOF]
  Demux1 : Demux  Outputs=[6;ROBOT_DOF]
  Discrete-Time Integrator : DiscreteIntegrator  InitialConditionSource=external  SampleTime=Ts  ICPrevOutput=DiscIntNeverNeededParam  ICPrevScaledInput=DiscIntNeverNeededParam
  Discrete-Time Integrator1 : DiscreteIntegrator  InitialConditionSource=external  SampleTime=Ts  ICPrevOutput=DiscIntNeverNeededParam  ICPrevScaledInput=DiscIntNeverNeededParam
  Mux : Mux  Inputs=2
  Terminator : Terminator
  floating base conversion : MATLAB Function  TreatAsAtomicUnit=on
  quatDerivative : Subsystem
  references : MATLAB Function  TreatAsAtomicUnit=on
  q_ikin : Outport
  inverseKinRef : Outport  Port=2
  Nu_ikin : Outport  Port=3
  wires:
  Nu_ikin_init/1 -> Discrete-Time Integrator/2
  q_ikin_init/1 -> Discrete-Time Integrator1/2
  dNu_ikin/1 -> Discrete-Time Integrator/1, references/1(dNu_ikin)
  Demux/2 -> Terminator/1
  Demux/1 -> quatDerivative/2(q_b)
  Discrete-Time Integrator1/1 -> references/3(q_ikin), Demux/1, floating base conversion/1(q_ikin_no_converted)
  Discrete-Time Integrator/1 -> Demux1/1, references/2(Nu_ikin), Nu_ikin/1
  Demux1/1 -> quatDerivative/1(omega_b)
  quatDerivative/1(dq_b) -> Mux/1
  Demux1/2 -> Mux/2
  Mux/1 -> Discrete-Time Integrator1/1
  references/1(inverseKinRef) -> inverseKinRef/1
  floating base conversion/1(q_ikin) -> q_ikin/1

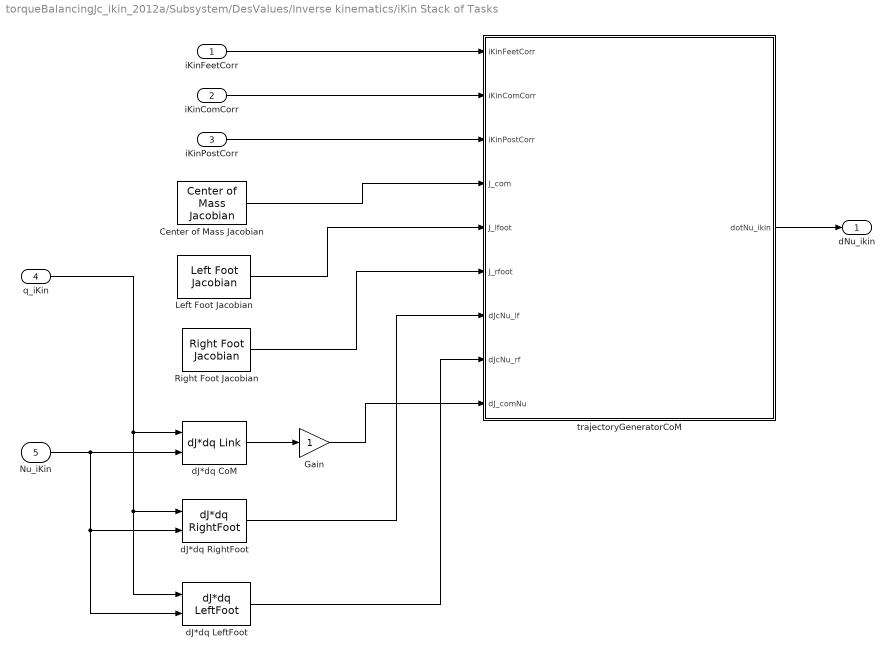
== system torqueBalancingJc_ikin_2012a/Subsystem/DesValues/Inverse kinematics/iKin Stack of Tasks ==
  iKinFeetCorr : Inport
  iKinComCorr : Inport  Port=2
  iKinPostCorr : Inport  Port=3
  q_iKin : Inport  Port=4
  Nu_iKin : Inport  Port=5
  Center of Mass Jacobian : WBCLibrary/wholeBodyModel/Jacobians/Center of Mass Jacobian  robotName=robotName  localName=localName
  Gain : Gain
  Left Foot Jacobian : WBCLibrary/wholeBodyModel/Jacobians/Left Foot Jacobian  robotName=robotName  localName=localName
  Right Foot Jacobian : WBCLibrary/wholeBodyModel/Jacobians/Right Foot Jacobian  robotName=robotName  localName=localName
  dJ*dq CoM : WBCLibrary/wholeBodyModel/Dynamics/dJ*dq Link  val=19  robotName=robotName  localName=localName  link=base
  dJ*dq LeftFoot : WBCLibrary/wholeBodyModel/Dynamics/dJ*dq LeftFoot  val=9  robotName=robotName  localName=localName
  dJ*dq RightFoot : WBCLibrary/wholeBodyModel/Dynamics/dJ*dq RightFoot  val=9  robotName=robotName  localName=localName
  trajectoryGeneratorCoM : MATLAB Function  TreatAsAtomicUnit=on
  dNu_ikin : Outport
  wires:
  trajectoryGeneratorCoM/1(dotNu_ikin) -> dNu_ikin/1
  Left Foot Jacobian/1 -> trajectoryGeneratorCoM/5(J_lfoot)
  Right Foot Jacobian/1 -> trajectoryGeneratorCoM/6(J_rfoot)
  iKinComCorr/1 -> trajectoryGeneratorCoM/2(iKinComCorr)
  iKinFeetCorr/1 -> trajectoryGeneratorCoM/1(iKinFeetCorr)
  iKinPostCorr/1 -> trajectoryGeneratorCoM/3(iKinPostCorr)
  Center of Mass Jacobian/1 -> trajectoryGeneratorCoM/4(J_com)
  q_iKin/1 -> dJ*dq LeftFoot/1, dJ*dq RightFoot/1, dJ*dq CoM/1
  Nu_iKin/1 -> dJ*dq LeftFoot/2, dJ*dq RightFoot/2, dJ*dq CoM/2
  dJ*dq CoM/1 -> Gain/1
  dJ*dq RightFoot/1 -> trajectoryGeneratorCoM/7(dJcNu_lf)
  dJ*dq LeftFoot/1 -> trajectoryGeneratorCoM/8(dJcNu_rf)
  Gain/1 -> trajectoryGeneratorCoM/9(dJ_comNu)

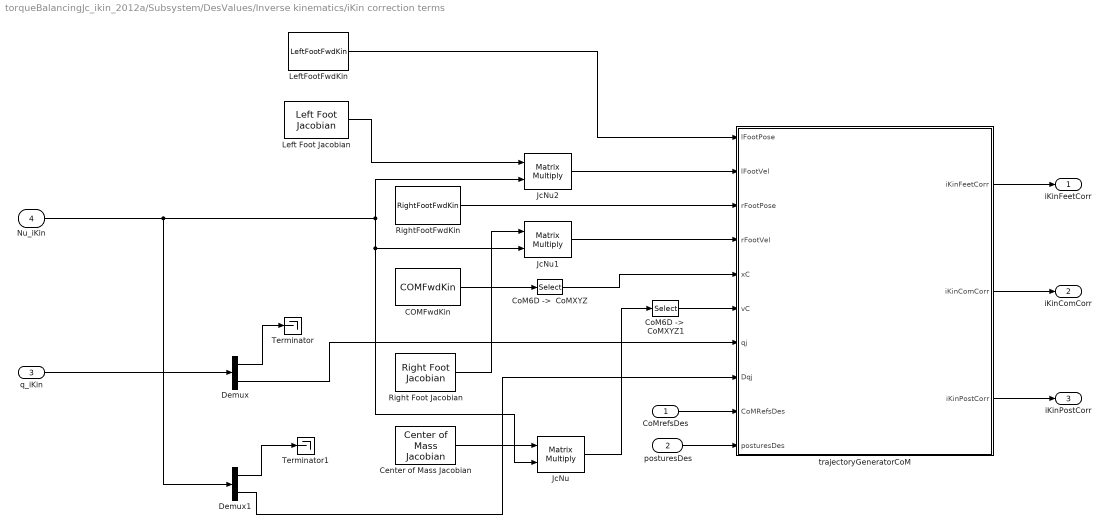
== system torqueBalancingJc_ikin_2012a/Subsystem/DesValues/Inverse kinematics/iKin correction terms ==
  CoMrefsDes : Inport
  posturesDes : Inport  Port=2
  q_iKin : Inport  Port=3
  Nu_iKin : Inport  Port=4
  "COMFwdKin " : WBCLibrary/wholeBodyModel/Forward Kinematics/COMFwdKin   robotName=robotName  localName=localName
  Center of Mass Jacobian : WBCLibrary/wholeBodyModel/Jacobians/Center of Mass Jacobian  robotName=robotName  localName=localName
  "CoM6D ->  CoMXYZ" : Selector  InputPortWidth=7  IndexOptions=Index vector (dialog)  Indices=[1 2 3]  OutputSizes=1
  "CoM6D ->  CoMXYZ1" : Selector  InputPortWidth=6  IndexOptions=Index vector (dialog)  Indices=[1 2 3]  OutputSizes=1
  Demux : Demux  Outputs=[16;ROBOT_DOF]
  Demux1 : Demux  Outputs=[6,ROBOT_DOF]
  JcNu : Product  Multiplication=Matrix(*)
  JcNu1 : Product  Multiplication=Matrix(*)
  JcNu2 : Product  Multiplication=Matrix(*)
  Left Foot Jacobian : WBCLibrary/wholeBodyModel/Jacobians/Left Foot Jacobian  robotName=robotName  localName=localName
  LeftFootFwdKin : WBCLibrary/wholeBodyModel/Forward Kinematics/LeftFootFwdKin  robotName=robotName  localName=localName
  Right Foot Jacobian : WBCLibrary/wholeBodyModel/Jacobians/Right Foot Jacobian  robotName=robotName  localName=localName
  RightFootFwdKin : WBCLibrary/wholeBodyModel/Forward Kinematics/RightFootFwdKin  robotName=robotName  localName=localName
  Terminator : Terminator
  Terminator1 : Terminator
  trajectoryGeneratorCoM : MATLAB Function  TreatAsAtomicUnit=on
  iKinFeetCorr : Outport
  iKinComCorr : Outport  Port=2
  iKinPostCorr : Outport  Port=3
  wires:
  trajectoryGeneratorCoM/1(iKinFeetCorr) -> iKinFeetCorr/1
  trajectoryGeneratorCoM/3(iKinPostCorr) -> iKinPostCorr/1
  trajectoryGeneratorCoM/2(iKinComCorr) -> iKinComCorr/1
  CoMrefsDes/1 -> trajectoryGeneratorCoM/9(CoMRefsDes)
  "COMFwdKin "/1 -> "CoM6D ->  CoMXYZ"/1
  "CoM6D ->  CoMXYZ"/1 -> trajectoryGeneratorCoM/5(xC)
  JcNu/1 -> "CoM6D ->  CoMXYZ1"/1
  posturesDes/1 -> trajectoryGeneratorCoM/10(posturesDes)
  "CoM6D ->  CoMXYZ1"/1 -> trajectoryGeneratorCoM/6(vC)
  JcNu1/1 -> trajectoryGeneratorCoM/4(rFootVel)
  RightFootFwdKin/1 -> trajectoryGeneratorCoM/3(rFootPose)
  JcNu2/1 -> trajectoryGeneratorCoM/2(lFootVel)
  Nu_iKin/1 -> Demux1/1, JcNu/2, JcNu1/2, JcNu2/2
  Left Foot Jacobian/1 -> JcNu2/1
  LeftFootFwdKin/1 -> trajectoryGeneratorCoM/1(lFootPose)
  q_iKin/1 -> Demux/1
  Right Foot Jacobian/1 -> JcNu1/1
  Center of Mass Jacobian/1 -> JcNu/1
  Demux1/2 -> trajectoryGeneratorCoM/8(Dqj)
  Demux/2 -> trajectoryGeneratorCoM/7(qj)
  Demux/1 -> Terminator/1
  Demux1/1 -> Terminator1/1

== system torqueBalancingJc_ikin_2012a/Subsystem/Dump and visualize/base + dq'/baseVelocity ==
  JacobRF : Inport
  JacobLF : Inport  Port=2
  dq : Inport  Port=3
  Constant : Constant  Value=LEFT_RIGHT_FOOT_IN_CONTACT
  MATLAB Function : MATLAB Function  TreatAsAtomicUnit=on
  baseVel : Outport
  wires:
  JacobLF/1 -> MATLAB Function/1(JcLeftFoot)
  JacobRF/1 -> MATLAB Function/2(JcRightFoot)
  MATLAB Function/1(y) -> baseVel/1
  dq/1 -> MATLAB Function/4(qD)
  Constant/1 -> MATLAB Function/3(activeFeetConstraints)

== system torqueBalancingJc_ikin_2012a/Subsystem/DesValues/Inverse kinematics/Integrator/quatDerivative ==
  omega_b : Inport
  q_b : Inport  Port=2
  quaternionDerivative : MATLAB Function  TreatAsAtomicUnit=on
  dq_b : Outport
  wires:
  omega_b/1 -> quaternionDerivative/1(dNu_b)
  quaternionDerivative/1(dot_qb) -> dq_b/1
  q_b/1 -> quaternionDerivative/2(q_b)

== matlab function Subsystem/M(q) h(q,dq) g(q)/fromFloating2Centroidal ==
  data: M input double; M_c output double; h input double; g input double; Jc input double; dJcNu input double; Nu input double; c_T_b input double; dT input double; h_c output double; Jc_c output double; Jc_cDNu_c output double; Nu_c output double
function [M_c,h_c, Jc_c, Jc_cDNu_c, Nu_c] = fromFloating2Centroidal(M, h, g, Jc, dJcNu, Nu, c_T_b, dT)
%#codegen
[M_c,C_cNu_c, g_c, Jc_c, Jc_cDNu_c, Nu_c] = fromFloatingToCentroidalDynamics(M, h, g, Jc, dJcNu, Nu, c_T_b, dT);
h_c = C_cNu_c + g_c;

== matlab function Subsystem/DesValues/trajectoryGeneratorCoM ==
  data: desired_x_dx_ddx_CoM output double; xCom0 input double; t input double; references parameter double
function desired_x_dx_ddx_CoM   = fcn(xCom0,t,references)
%#codegen
        
if t > references.noOscillationTime
    A = references.amplitudeOfOscillation;
else
    A = 0;
end
f = references.frequencyOfOscillation;

xcomDes    = xCom0 + A*sin(2*pi*f*t)*references.directionOfOscillation;
% xcomDes(1) =  xcomDes(1) + 0.01;
xDcomDes   =         A*2*pi*f*cos(2*pi*f*t)*references.directionOfOscillation;
xDDcomDes  =        -A*(2*pi*f)^2*sin(2*pi*f*t)*references.directionOfOscillation;

desired_x_dx_ddx_CoM = [xcomDes;xDcomDes;xDDcomDes];

== matlab function Subsystem/emergency stop: joint limits/MATLAB Function ==
  data: umin input double; umax input double; u input double; inRange output double; tol input double
function inRange = checkRange(umin, umax, u, tol)
%#codegen

res = u < umin + tol | u > umax - tol;
res = sum(res);
if res==0
    inRange = 1;
else
    inRange = 0;
    u < umin + tol | u > umax - tol
end

== matlab function Subsystem/controller_QP/tau(f)  ==
  data: tau output double; constraints input double; ROBOT_DOF_FOR_SIMULINK input double; ConstraintsMatrix input double; bVectorConstraints input double; qj input double; Nu input double; inverseKinRef input double; M input double; h input double; Jc input double; JcDNu input double; impedances input double; reg parameter double; gain parameter double; fc output double
function [tau,fc]    =  controller(constraints,ROBOT_DOF_FOR_SIMULINK,ConstraintsMatrix,bVectorConstraints,qj,Nu,inverseKinRef, M,h , Jc, JcDNu, impedances,reg,gain)
%#codegen

ROBOT_DOF = size(ROBOT_DOF_FOR_SIMULINK,1);

qTilde    = qj - inverseKinRef(:,1);
qTildeD   = Nu(7:end) - inverseKinRef(:,2);
qDesDD    = inverseKinRef(:,3);
[tau,fc]       = controllerFCN(constraints, ROBOT_DOF, M, h, Jc, JcDNu,impedances, gain.dampings, qTilde,qTildeD, qDesDD,reg);

== matlab function Subsystem/M(q) h(q,dq) g(q)/fromState2TandTD ==
  data: M input double; xcom input double; c_T_b output double; wHb input double; dxcom input double; dx_b input double; dT output double
function [c_T_b, dT] = centroidalTransformationT_TDot(M,xcom,wHb,dxcom,dx_b)
%#codegen
[c_T_b, dT] = centroidalTransformationT_TDot(xcom,wHb(1:3,4),dxcom,dx_b,M);

== matlab function Subsystem/Dump and visualize/base + dq'/baseVelocity/MATLAB Function ==
  data: JcLeftFoot input double; JcRightFoot input double; activeFeetConstraints input double; y output double; qD input double
function y = fcn(JcLeftFoot,JcRightFoot,activeFeetConstraints,qD)
%#codegen
if sum(activeFeetConstraints) == 2
    Jc = [JcLeftFoot;JcRightFoot];
else
    Jc = JcLeftFoot;
end
y = -pinv(Jc(:,1:6))*Jc(:,7:end)*qD;

== matlab function Subsystem/nonlinearImpedances/nonlinearPosturalGains  ==
  data: qDes input double; nonlinearImpedences output double; q input double; qMin input double; qMax input double; gain parameter double
function nonlinearImpedences = fcn(qDes,q,qMin,qMax,gain)
    %#codegen
    qDes = qDes(:,1);
    impedences_at_0     = gain.impedances;
    increasingRatesImp  = (gain.increasingRatesImp)';
    qTildeMax           = gain.qTildeMax;

    tp =  pi./(2*(qMax-qDes));
    tn = -pi./(2*(qMin-qDes));

    
    qTilde = q - qDes;
            
    nonlinearImpedences = (impedences_at_0'   + increasingRatesImp.*tan(pi.*qTilde./(2*qTildeMax)).^2)';
%                                               increasingRatesImp.*tan((tp.*stepFcn(qTilde) + tn.*stepFcn(-qTilde)).*qTilde).^2)';
                                           
end

function y = stepFcn(x) 
   %#codegen
   y = x > 0; 
end

== matlab function Subsystem/M(q) h(q,dq) g(q)/composingSmoothJacobians ==
  data: constraints input double; JL input double; JR input double; Jc output double; JLNuD input double; JRNuD input double; JcDNuD output double
function [Jc, JcDNuD] = composingSmoothJacobians(constraints,JL,JR, JLNuD,JRNuD)
%#codegen
Jc     = [ JL*constraints(1) ;
           JR*constraints(2)];
       
JcDNuD = [ JLNuD*constraints(1) ;
           JRNuD*constraints(2)];

== matlab function Subsystem/set Base velocity/baseVelocity/MATLAB Function ==
  data: JcLeftFoot input double; JcRightFoot input double; activeFeetConstraints input double; y output double; qD input double; reg parameter double
function y = fcn(JcLeftFoot,JcRightFoot,activeFeetConstraints,qD,reg)
%#codegen

Jc = [ JcLeftFoot*activeFeetConstraints(1);
      JcRightFoot*activeFeetConstraints(2)];

Jcj =  Jc(:,1:6);
pinvJcj = (Jcj')/(Jcj*Jcj' + reg.pinvDamp*eye(size(Jcj,1)));
  
% pinvJcj = pinv(Jc(:,1:6));

y = -pinvJcj*Jc(:,7:end)*qD;

== matlab function Subsystem/DesValues/Inverse kinematics/Integrator/quatDerivative/quaternionDerivative ==
  data: dNu_b input double; dot_qb output double; q_b input double
function dot_qb   = fcn( dNu_b, q_b )

%apply the conversion of reference frame between base and wolrd
omega_b        = dNu_b(4:end);

[~,dcm]        = frame2posrot(q_b);

omega_w        = (dcm')*omega_b;

%calculate the quaternion derivative
quat_base      = q_b(4:end);

dot_qb_b         = quaternionDerivative( omega_w, quat_base );

dot_qb = [dNu_b(1:3);dot_qb_b];

end

== matlab function Subsystem/DesValues/Inverse kinematics/Integrator/references ==
  data: dNu_ikin input double; inverseKinRef output double; Nu_ikin input double; q_ikin input double
function inverseKinRef = fcn(dNu_ikin, Nu_ikin, q_ikin)
%#codegen

%composing the joint reference 
ddq_j_ref = dNu_ikin(7:end);
dq_j_ref  = Nu_ikin(7:end);
q_j_ref   = q_ikin(8:end);


inverseKinRef = [q_j_ref dq_j_ref ddq_j_ref];

== matlab function Subsystem/DesValues/Inverse kinematics/Integrator/floating base conversion ==
  data: q_ikin_no_converted input double; q_ikin output double
function q_ikin = fcn(q_ikin_no_converted)
%#codegen

% define the rototraslation matrix
q_b = q_ikin_no_converted(1:7);

[pos,rot] = frame2posrot(q_b);

Rototr_b  = [rot pos; [0 0 0 1]]';

% row-major serialization
vect_R    = Rototr_b(:);
% vect_R  = zeros(16,1);

%new state vector
q_ikin    = [vect_R; q_ikin_no_converted(8:end)];

end

== matlab function Subsystem/DesValues/Inverse kinematics/iKin Stack of Tasks/trajectoryGeneratorCoM ==
  data: iKinFeetCorr input double; iKinComCorr input double; iKinPostCorr input double; J_com input double; J_lfoot input double; J_rfoot input double; dotNu_ikin output double; dJcNu_lf input double; dJcNu_rf input double; dJ_comNu input double
function dotNu_ikin   = fcn(iKinFeetCorr, iKinComCorr, iKinPostCorr, J_com, J_lfoot, J_rfoot,dJcNu_lf, dJcNu_rf, dJ_comNu)
%#codegen
n_joints = size(J_com(:,7:end),2);

%% jacobians and their derivatives
Jc   = [J_lfoot ; J_rfoot];
Jcom = J_com(1:3,:);
Jp   = [zeros(n_joints,6),eye(n_joints)]; 

dJcNu   = [dJcNu_lf; dJcNu_rf];
dJcomNu = dJ_comNu(1:3);

%% state acceleration reference calculation
dotNu_ikin   = Ikin_AccelerationRef_generator(Jc, Jcom, Jp, dJcNu, dJcomNu,iKinFeetCorr, iKinComCorr, iKinPostCorr); 

end

== matlab function Subsystem/DesValues/Inverse kinematics/iKin correction terms/trajectoryGeneratorCoM ==
  data: lFootPose input double; lFootVel input double; rFootPose input double; rFootVel input double; xC input double; vC input double; qj input double; Dqj input double; iKinFeetCorr output double; CoMRefsDes input double; iKinComCorr output double; iKinPostCorr output double; posturesDes input double; gain parameter double
function [iKinFeetCorr,iKinComCorr,iKinPostCorr]  = fcn(lFootPose,lFootVel,rFootPose,rFootVel,xC,vC,qj,Dqj,CoMRefsDes,posturesDes,gain)
%#codegen

iKinFeetCorr = [-gain.ikin.kp*lFootPose(1:3)-gain.ikin.kd*lFootVel(1:3);
                                            -gain.ikin.kd*lFootVel(4:6);
              -0*gain.ikin.kp*rFootPose(1:3)-gain.ikin.kd*rFootVel(1:3);
                                            -gain.ikin.kd*rFootVel(4:6)];
                                         
iKinComCorr  = CoMRefsDes(:,3)-gain.ikin.kp*(xC-CoMRefsDes(:,1))-gain.ikin.kd*(vC-CoMRefsDes(:,2));

iKinPostCorr = posturesDes(:,3)-gain.ikin.kp*(qj-posturesDes(:,1))-gain.ikin.kd*(Dqj-posturesDes(:,2));
